simulink model "Fixed_time_NN"  (R2019b)
settings: Solver=ode4  StartTime=0.0  StopTime=10.0  FixedStep=0.001  RelTol=1e-3
settings Model: Creator=xyh  LastModifiedBy=user
settings DataIOCC: ReturnWorkspaceOutputs=off

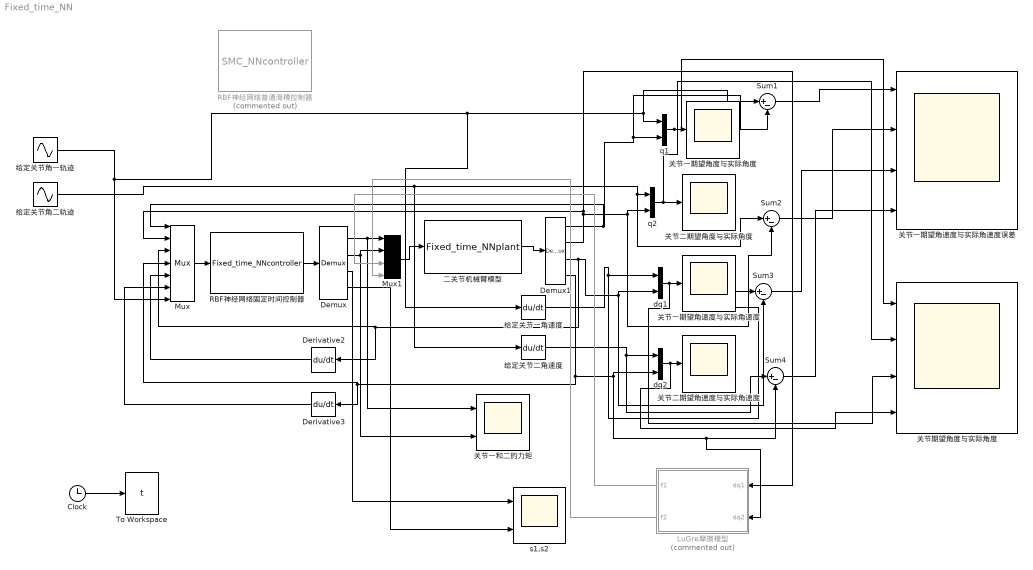
== system Fixed_time_NN ==
  Clock : Clock
  Demux : Demux
  Demux1 : Demux
  Derivative2 : Derivative
  Derivative3 : Derivative
  LuGre摩擦模型 : Subsystem  Commented=on
  Mux : Mux  Inputs=7
  Mux1 : Mux
  RBF神经网络固定时间控制器 : S-Function  FunctionName=Fixed_time_NNcontroller  SFunctionDeploymentMode=off  EnableBusSupport=off
  RBF神经网络普通滑模控制器 : S-Function  Commented=on  FunctionName=SMC_NNcontroller  SFunctionDeploymentMode=off  EnableBusSupport=off
  Sum{1..4} (4 alike) : Sum  Inputs=|+-
  To Workspace : ToWorkspace  VariableName=t  SampleTime=-1
  dq1 : Mux  Inputs=2
  dq2 : Mux  Inputs=2
  q1 : Mux  Inputs=2
  q2 : Mux  Inputs=2
  s1,s2 : Scope  NumInputPorts=2
  二关节机械臂模型 : S-Function  FunctionName=Fixed_time_NNplant  SFunctionDeploymentMode=off  EnableBusSupport=off
  关节一和二的力矩 : Scope  NumInputPorts=2
  关节一期望角度与实际角度 : Scope
  关节一期望角速度与实际角速度 : Scope
  关节一期望角速度与实际角速度误差 : Scope  NumInputPorts=4
  关节二期望角度与实际角度 : Scope
  关节二期望角速度与实际角速度 : Scope
  关节期望角度与实际角度 : Scope  NumInputPorts=4
  给定关节一角速度 : Derivative
  给定关节二角速度 : Derivative
  给定关节角一轨迹 : Sin  Amplitude=0.5  Frequency=pi  SampleTime=0
  给定关节角二轨迹 : Sin  Amplitude=0.5  Frequency=pi  SampleTime=0
  wires:
  Demux/4 -> s1,s2/2
  给定关节角二轨迹/1 -> q2/1, Sum2/1, 给定关节二角速度/1
  Sum4/1 -> 关节一期望角速度与实际角速度误差/4
  Sum3/1 -> 关节一期望角速度与实际角速度误差/3
  Demux/3 -> s1,s2/1
  Sum1/1 -> 关节一期望角速度与实际角速度误差/1
  Derivative3/1 -> Mux/6
  Demux1/2 -> LuGre摩擦模型/1(dq1), Mux/2, Sum2/2, q2/2
  RBF神经网络固定时间控制器/1 -> Demux/1
  Demux/2 -> 关节一和二的力矩/2, Mux1/2
  Sum2/1 -> 关节一期望角速度与实际角速度误差/2
  给定关节角一轨迹/1 -> Mux/7, 给定关节一角速度/1, q1/1, Sum1/1
  Derivative2/1 -> Mux/5
  给定关节二角速度/1 -> Sum4/1, dq2/1
  Demux/1 -> 关节一和二的力矩/1, Mux1/1
  Clock/1 -> To Workspace/1
  Demux1/3 -> Mux/3, Derivative2/1, Sum3/2, dq1/2
  Demux1/4 -> LuGre摩擦模型/2(dq2), Sum4/2, dq2/2, Mux/4, Derivative3/1
  给定关节一角速度/1 -> dq1/1, Sum3/1
  Mux1/1 -> 二关节机械臂模型/1
  Mux/1 -> RBF神经网络固定时间控制器/1
  Demux1/1 -> Mux/1, q1/2, Sum1/2
  二关节机械臂模型/1 -> Demux1/1
  q1/1 -> 关节期望角度与实际角度/1, 关节一期望角度与实际角度/1
  q2/1 -> 关节期望角度与实际角度/2, 关节二期望角度与实际角度/1
  dq1/1 -> 关节期望角度与实际角度/3, 关节一期望角速度与实际角速度/1
  dq2/1 -> 关节期望角度与实际角度/4, 关节二期望角速度与实际角速度/1
  LuGre摩擦模型/1(f1) -> Mux1/3
  LuGre摩擦模型/2(f2) -> Mux1/4

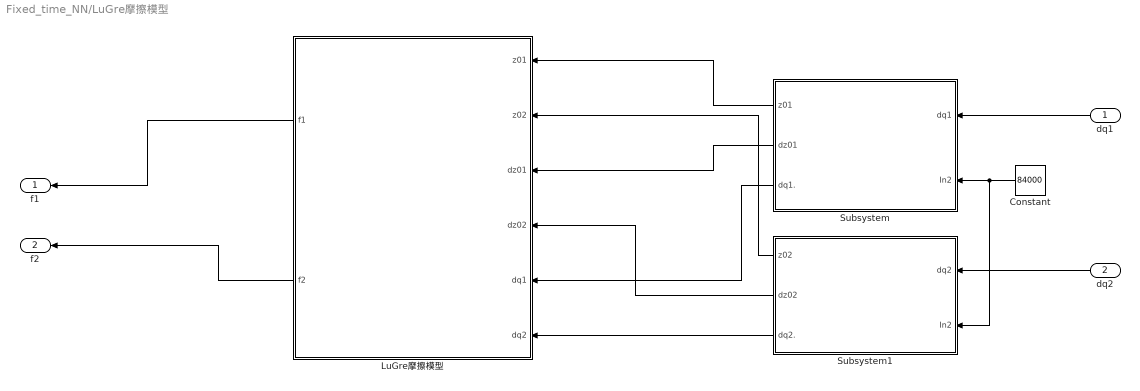
== system Fixed_time_NN/LuGre摩擦模型 ==
  dq1 : Inport
  dq2 : Inport  Port=2
  Constant : Constant  Value=84000
  LuGre摩擦模型 : MATLAB Function  TreatAsAtomicUnit=on
  Subsystem : Subsystem
  Subsystem1 : Subsystem
  f1 : Outport
  f2 : Outport  Port=2
  wires:
  LuGre摩擦模型/2(f2) -> f2/1
  LuGre摩擦模型/1(f1) -> f1/1
  Constant/1 -> Subsystem1/2(In2), Subsystem/2(In2)
  dq1/1 -> Subsystem/1(dq1)
  Subsystem/1(z01) -> LuGre摩擦模型/1(z01)
  Subsystem/2(dz01) -> LuGre摩擦模型/3(dz01)
  Subsystem/3(dq1.) -> LuGre摩擦模型/5(dq1)
  dq2/1 -> Subsystem1/1(dq2)
  Subsystem1/1(z02) -> LuGre摩擦模型/2(z02)
  Subsystem1/2(dz02) -> LuGre摩擦模型/4(dz02)
  Subsystem1/3(dq2.) -> LuGre摩擦模型/6(dq2)

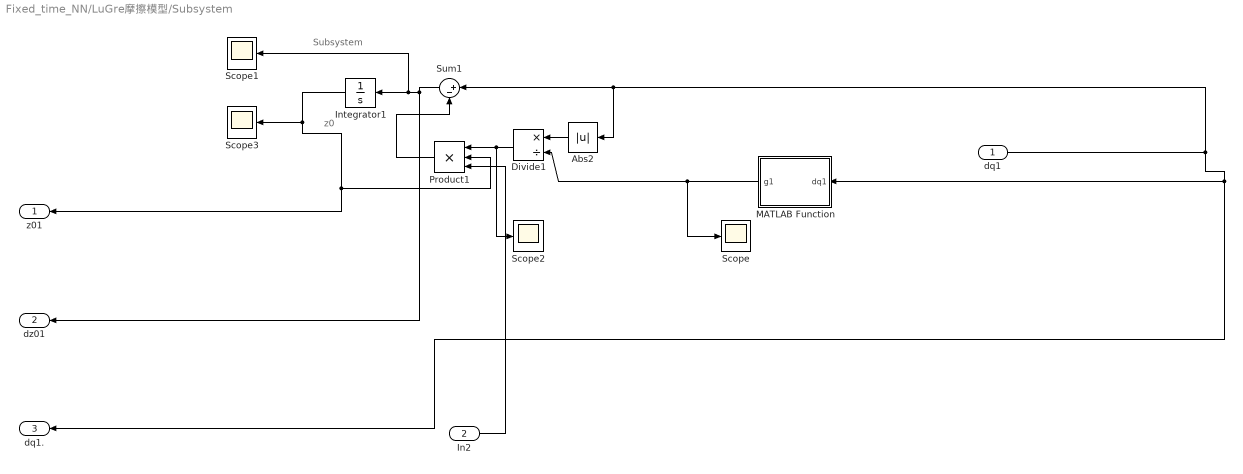
== system Fixed_time_NN/LuGre摩擦模型/Subsystem ==
  note: z0
  note: Subsystem
  dq1 : Inport
  In2 : Inport  Port=2
  Abs2 : Abs
  Divide1 : Product  Inputs=*/
  Integrator1 : Integrator
  MATLAB Function : MATLAB Function  TreatAsAtomicUnit=on
  Product1 : Product  Inputs=3
  Scope{,1..3} (4 alike) : Scope
  Sum1 : Sum  Inputs=|+-
  z01 : Outport
  dz01 : Outport  Port=2
  dq1. : Outport  Port=3
  wires:
  Product1/1 -> Sum1/2
  Abs2/1 -> Divide1/1
  Integrator1/1 -> Scope3/1, z01/1, Product1/2
  Sum1/1 -> dz01/1, Scope1/1, Integrator1/1
  Divide1/1 -> Product1/1, Scope2/1
  dq1/1 -> Abs2/1, Sum1/1, dq1./1, MATLAB Function/1(dq1)
  In2/1 -> Product1/3
  MATLAB Function/1(g1) -> Divide1/2, Scope/1

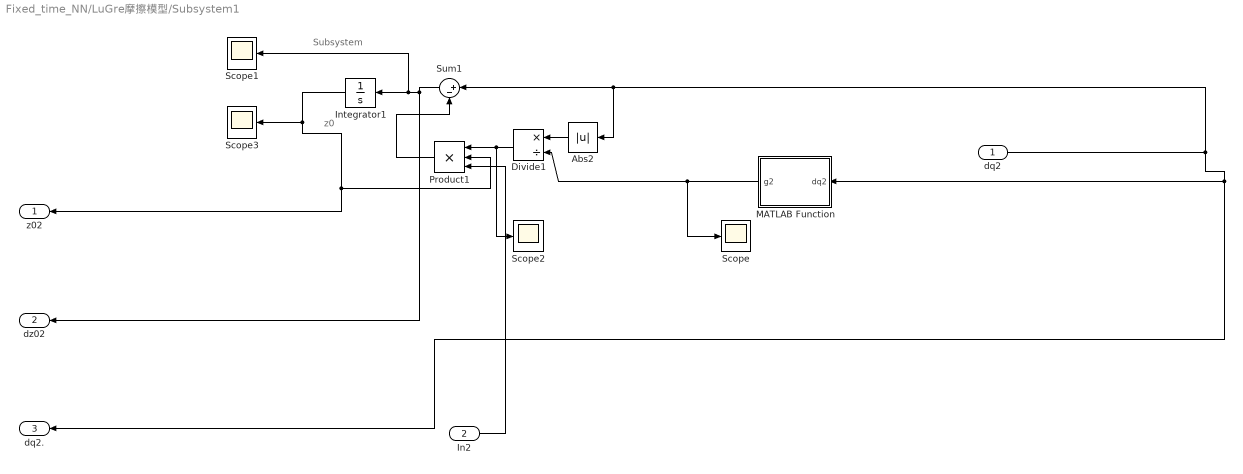
== system Fixed_time_NN/LuGre摩擦模型/Subsystem1 ==
  note: Subsystem
  note: z0
  dq2 : Inport
  In2 : Inport  Port=2
  Abs2 : Abs
  Divide1 : Product  Inputs=*/
  Integrator1 : Integrator
  MATLAB Function : MATLAB Function  TreatAsAtomicUnit=on
  Product1 : Product  Inputs=3
  Scope{,1..3} (4 alike) : Scope
  Sum1 : Sum  Inputs=|+-
  z02 : Outport
  dz02 : Outport  Port=2
  dq2. : Outport  Port=3
  wires:
  MATLAB Function/1(g2) -> Scope/1, Divide1/2
  In2/1 -> Product1/3
  dq2/1 -> MATLAB Function/1(dq2), dq2./1, Sum1/1, Abs2/1
  Divide1/1 -> Scope2/1, Product1/1
  Sum1/1 -> Integrator1/1, Scope1/1, dz02/1
  Integrator1/1 -> Product1/2, z02/1, Scope3/1
  Abs2/1 -> Divide1/1
  Product1/1 -> Sum1/2

== matlab function Fixed_time_NN/LuGre摩擦模型/Subsystem1/MATLAB Function ==
  data: dq2 input; g2 output
function g2 = fcn(dq2)
xite1 = 260;
xite2 = 28;
Fc = 3.82;
Fs = 8.16;
dqs = 0.0125;

g2 = Fc + (Fs-Fc)*exp(-(dq2/dqs)^2);

== matlab function Fixed_time_NN/LuGre摩擦模型/LuGre摩擦模型 ==
  data: z01 input; z02 input; dz01 input; dz02 input; dq1 input; f1 output; dq2 input; f2 output
function [f1,f2] = fcn(z01,z02,dz01,dz02,dq1,dq2)
xite0 = 84000;
xite1 = 260;
xite2 = 28;
Fc = 3.82;
Fs = 8.16;
dqs = 0.0125;
lamda = 1;

f1 = lamda * (xite0 * z01 + xite1 * dz01 + xite2 * dq1);
f2 = lamda * (xite0 * z02 + xite1 * dz02 + xite2 * dq2);

== matlab function Fixed_time_NN/LuGre摩擦模型/Subsystem/MATLAB Function ==
  data: dq1 input; g1 output
function g1 = fcn(dq1)
xite1 = 260;
xite2 = 28;
Fc = 3.82;
Fs = 8.16;
dqs = 0.0125;

g1 = Fc + (Fs-Fc)*exp(-(dq1/dqs)^2);
